simulink model "modelo_completo"  (R2017b)
settings: Solver=VariableStepAuto  StartTime=0.0  StopTime=5  RelTol=1e-3
libraries: simulink x5
settings Model: Creator=jorgeluis  LastModifiedBy=jorgeluis

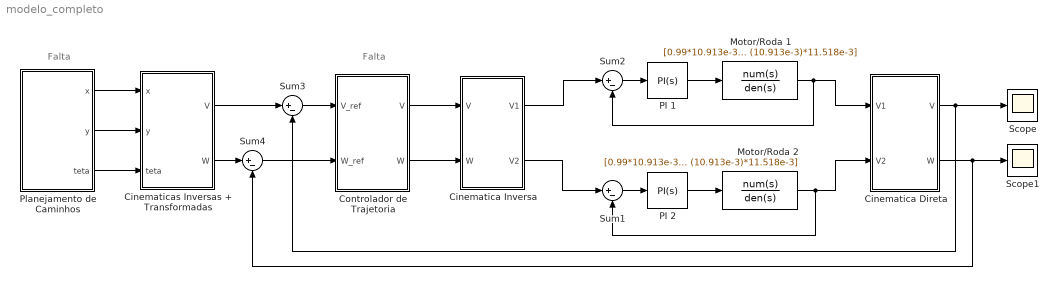
== system modelo_completo ==
  note: Falta
  note: Falta
  Cinematica Direta : Subsystem
  Cinematica Inversa : Subsystem
  Cinematicas Inversas + Transformadas : Subsystem
  Controlador de Trajetoria : Subsystem
  Motor/Roda 1 : TransferFcn  Numerator=[0.99*10.913e-3]  Denominator=[(1.5506*9.35604e-3) (10.913e-3)*11.518e-3]
  Motor/Roda 2 : TransferFcn  Numerator=[0.99*10.913e-3]  Denominator=[(1.5506*9.35604e-3) (10.913e-3)*11.518e-3]
  PI 1 : simulink/Continuous/PID Controller  Controller=PI  TimeDomain=Continuous-time  SampleTime=-1  IntegratorMethod=Forward Euler  FilterMethod=Forward Euler  Form=Ideal  UseFilter=on  ControllerParametersSource=internal  P=1.0800  I=0.0433  D=0  N=0  InitialConditionSource=internal  InitialConditionForIntegrator=0  InitialConditionForFilter=0  ExternalReset=none  LimitOutput=off  UpperSaturationLimit=inf  LowerSaturationLimit=-inf  LinearizeAsGain=on  AntiWindupMode=none  Kb=1  TrackingMode=off  Kt=1  PParamMin=[]  PParamMax=[]  IParamMin=[]  IParamMax=[]  DParamMin=[]  DParamMax=[]  NParamMin=[]  NParamMax=[]  KbParamMin=[]  KbParamMax=[]  KtParamMin=[]  KtParamMax=[]  POutMin=[]  POutMax=[]  IOutMin=[]  IOutMax=[]  DOutMin=[]  DOutMax=[]  NOutMin=[]  NOutMax=[]  KbOutMin=[]  KbOutMax=[]  KtOutMin=[]  KtOutMax=[]  IntegratorOutMin=[]  IntegratorOutMax=[]  FilterOutMin=[]  FilterOutMax=[]  SumOutMin=[]  SumOutMax=[]  SumI1OutMin=[]  SumI1OutMax=[]  SumI2OutMin=[]  SumI2OutMax=[]  SumI3OutMin=[]  SumI3OutMax=[]  SumDOutMin=[]  SumDOutMax=[]  SaturationOutMin=[]  SaturationOutMax=[]  IntegratorContinuousStateAttributes=''  IntegratorStateMustResolveToSignalObject=off  IntegratorRTWStateStorageClass=Auto  FilterContinuousStateAttributes=''  FilterStateMustResolveToSignalObject=off  FilterRTWStateStorageClass=Auto  DifferentiatorICPrevScaledInput=0  DifferentiatorOutMin=[]  DifferentiatorOutMax=[]  InitialConditionSetting=State (most efficient)  FilterDiffOutCoefMin=[]  FilterDiffOutCoefMax=[]  SumDenOutMin=[]  SumDenOutMax=[]  SumNumOutMin=[]  SumNumOutMax=[]  ReciprocalOutMin=[]  ReciprocalOutMax=[]  DivideOutMin=[]  DivideOutMax=[]  TunerSelectOption=Transfer Function Based (PID Tuner App)
  PI 2 : simulink/Continuous/PID Controller  Controller=PI  TimeDomain=Continuous-time  SampleTime=-1  IntegratorMethod=Forward Euler  FilterMethod=Forward Euler  Form=Ideal  UseFilter=on  ControllerParametersSource=internal  P=1.0800  I=0.0433  D=0  N=0  InitialConditionSource=internal  InitialConditionForIntegrator=0  InitialConditionForFilter=0  ExternalReset=none  LimitOutput=off  UpperSaturationLimit=inf  LowerSaturationLimit=-inf  LinearizeAsGain=on  AntiWindupMode=none  Kb=1  TrackingMode=off  Kt=1  PParamMin=[]  PParamMax=[]  IParamMin=[]  IParamMax=[]  DParamMin=[]  DParamMax=[]  NParamMin=[]  NParamMax=[]  KbParamMin=[]  KbParamMax=[]  KtParamMin=[]  KtParamMax=[]  POutMin=[]  POutMax=[]  IOutMin=[]  IOutMax=[]  DOutMin=[]  DOutMax=[]  NOutMin=[]  NOutMax=[]  KbOutMin=[]  KbOutMax=[]  KtOutMin=[]  KtOutMax=[]  IntegratorOutMin=[]  IntegratorOutMax=[]  FilterOutMin=[]  FilterOutMax=[]  SumOutMin=[]  SumOutMax=[]  SumI1OutMin=[]  SumI1OutMax=[]  SumI2OutMin=[]  SumI2OutMax=[]  SumI3OutMin=[]  SumI3OutMax=[]  SumDOutMin=[]  SumDOutMax=[]  SaturationOutMin=[]  SaturationOutMax=[]  IntegratorContinuousStateAttributes=''  IntegratorStateMustResolveToSignalObject=off  IntegratorRTWStateStorageClass=Auto  FilterContinuousStateAttributes=''  FilterStateMustResolveToSignalObject=off  FilterRTWStateStorageClass=Auto  DifferentiatorICPrevScaledInput=0  DifferentiatorOutMin=[]  DifferentiatorOutMax=[]  InitialConditionSetting=State (most efficient)  FilterDiffOutCoefMin=[]  FilterDiffOutCoefMax=[]  SumDenOutMin=[]  SumDenOutMax=[]  SumNumOutMin=[]  SumNumOutMax=[]  ReciprocalOutMin=[]  ReciprocalOutMax=[]  DivideOutMin=[]  DivideOutMax=[]  TunerSelectOption=Transfer Function Based (PID Tuner App)
  Planejamento de Caminhos : Subsystem
  Scope : Scope
  Scope1 : Scope
  Sum{1..4} (4 alike) : Sum  Inputs=|+-
  wires:
  Sum1/1 -> PI 2/1
  PI 2/1 -> Motor/Roda 2/1
  PI 1/1 -> Motor/Roda 1/1
  Sum2/1 -> PI 1/1
  Cinematica Inversa/1(V1) -> Sum2/1
  Cinematica Inversa/2(V2) -> Sum1/1
  Motor/Roda 1/1 -> Sum2/2, Cinematica Direta/1(V1)
  Motor/Roda 2/1 -> Sum1/2, Cinematica Direta/2(V2)
  Controlador de Trajetoria/1(V) -> Cinematica Inversa/1(V)
  Controlador de Trajetoria/2(W) -> Cinematica Inversa/2(W)
  Cinematica Direta/1(V) -> Scope/1, Sum3/2
  Cinematica Direta/2(W) -> Scope1/1, Sum4/2
  Sum3/1 -> Controlador de Trajetoria/1(V_ref)
  Sum4/1 -> Controlador de Trajetoria/2(W_ref)
  Cinematicas Inversas + Transformadas/2(W) -> Sum4/1
  Cinematicas Inversas + Transformadas/1(V) -> Sum3/1
  Planejamento de Caminhos/1(x) -> Cinematicas Inversas + Transformadas/1(x)
  Planejamento de Caminhos/2(y) -> Cinematicas Inversas + Transformadas/2(y)
  Planejamento de Caminhos/3(teta) -> Cinematicas Inversas + Transformadas/3(teta)

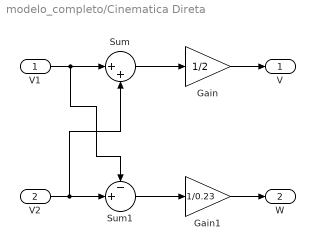
== system modelo_completo/Cinematica Direta ==
  V1 : Inport
  V2 : Inport  Port=2
  Gain : Gain  Gain=1/2
  Gain1 : Gain  Gain=1/0.23
  Sum : Sum  Inputs=|++
  Sum1 : Sum  Inputs=-+|
  V : Outport
  W : Outport  Port=2
  wires:
  V2/1 -> Sum/2, Sum1/2
  V1/1 -> Sum1/1, Sum/1
  Sum/1 -> Gain/1
  Gain1/1 -> W/1
  Gain/1 -> V/1
  Sum1/1 -> Gain1/1

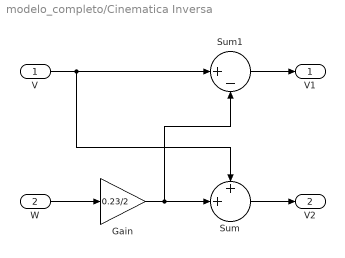
== system modelo_completo/Cinematica Inversa ==
  V : Inport
  W : Inport  Port=2
  Gain : Gain  Gain=0.23/2
  Sum : Sum  Inputs=++|
  Sum1 : Sum  Inputs=|+-
  V1 : Outport
  V2 : Outport  Port=2
  wires:
  W/1 -> Gain/1
  Sum1/1 -> V1/1
  Gain/1 -> Sum1/2, Sum/2
  V/1 -> Sum/1, Sum1/1
  Sum/1 -> V2/1

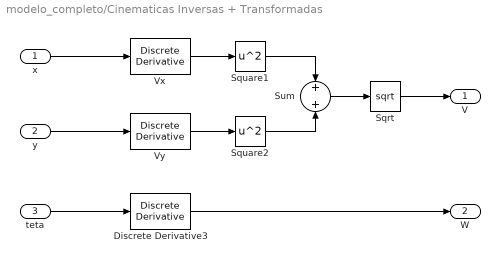
== system modelo_completo/Cinematicas Inversas + Transformadas ==
  x : Inport
  y : Inport  Port=2
  teta : Inport  Port=3
  Discrete Derivative3 : simulink/Discrete/Discrete Derivative  gainval=1.0  ICPrevScaledInput=0.0  OutMin=[]  OutMax=[]  OutDataType=fixdt(1, 16)  OutScaling=2^-10  DoSatur=off
  Sqrt : Sqrt  SaturateOnIntegerOverflow=on
  Square1 : Math  Operator=square  RndMeth=Zero  SaturateOnIntegerOverflow=on
  Square2 : Math  Operator=square  RndMeth=Zero  SaturateOnIntegerOverflow=on
  Sum : Sum  Inputs=+|+
  Vx : simulink/Discrete/Discrete Derivative  gainval=1.0  ICPrevScaledInput=0.0  OutMin=[]  OutMax=[]  OutDataType=fixdt(1, 16)  OutScaling=2^-10  DoSatur=off
  Vy : simulink/Discrete/Discrete Derivative  gainval=1.0  ICPrevScaledInput=0.0  OutMin=[]  OutMax=[]  OutDataType=fixdt(1, 16)  OutScaling=2^-10  DoSatur=off
  V : Outport
  W : Outport  Port=2
  wires:
  Discrete Derivative3/1 -> W/1
  teta/1 -> Discrete Derivative3/1
  x/1 -> Vx/1
  Sqrt/1 -> V/1
  y/1 -> Vy/1
  Vx/1 -> Square1/1
  Vy/1 -> Square2/1
  Square1/1 -> Sum/1
  Square2/1 -> Sum/2
  Sum/1 -> Sqrt/1

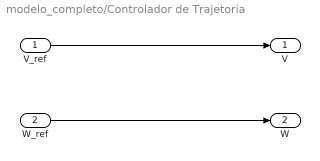
== system modelo_completo/Controlador de Trajetoria ==
  V_ref : Inport
  W_ref : Inport  Port=2
  V : Outport
  W : Outport  Port=2
  wires:
  V_ref/1 -> V/1
  W_ref/1 -> W/1

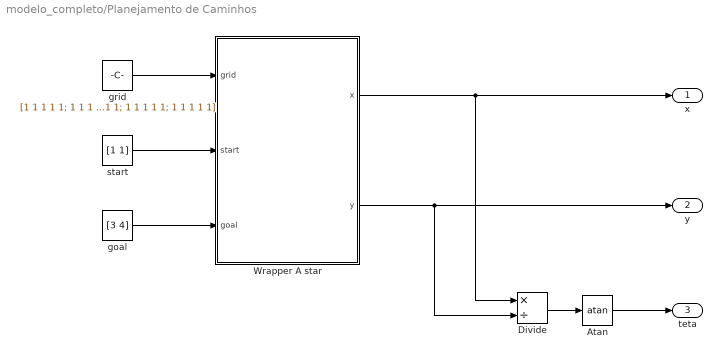
== system modelo_completo/Planejamento de Caminhos ==
  Atan : Trigonometry  Operator=atan
  Divide : Product  Inputs=*/
  Wrapper A star : MATLAB Function  TreatAsAtomicUnit=on
  goal : Constant  Value=[3 4]
  grid : Constant  Value=[1 1 1 1 1; 1 1 1 1 1; 1 1 1 1 1; 1 1 1 1 1; 1 1 1 1 1]
  start : Constant  Value=[1 1]
  x : Outport
  y : Outport  Port=2
  teta : Outport  Port=3
  wires:
  Wrapper A star/1(x) -> Divide/1, x/1
  Wrapper A star/2(y) -> Divide/2, y/1
  Atan/1 -> teta/1
  grid/1 -> Wrapper A star/1(grid)
  Divide/1 -> Atan/1
  start/1 -> Wrapper A star/2(start)
  goal/1 -> Wrapper A star/3(goal)

== matlab function modelo_completo/Planejamento de Caminhos/Wrapper A star ==
  data: grid input; start input; x output size=1 [0..1000]; goal input; y output size=1 [0..1000]
% Autores: Jorgeluis Guerra
%          Luis Braga
%          Saulo Alves

% Funcao wrapper que insere o algoritmo do A estrela dentro do modelo do
% robo

function [x, y] = wrapper_a_star(grid, start, goal)

   % Valor 'infinito'
   INF = 100000;
   % Limites do grid de celulas
   GRID_MIN = 1;
   GRID_MAX = 5;

   start_node.x = start(1);
   start_node.y = start(2);
   start_node.g = INF;
   start_node.f = INF;
   start_node.camefrom = [];

   goal_node.x = goal(1);
   goal_node.y = goal(2);
   goal_node.g = INF;
   goal_node.f = INF;
   goal_node.camefrom = [];

   path_nodes = a_star(start_node, goal_node);

   for i = path_nodes
      x = i.x;
      y = i.y;
   end
end
